simulink model "TwoDegreeFreedom_Model"  (R2019a)
settings: Solver=VariableStepAuto  StartTime=0.0  StopTime=10.0  RelTol=1e-3
undefined symbols (not defined in the file): C_s, K_s, K_t, m_s, m_u
settings Model: Creator=ansar  LastModifiedBy=ansar

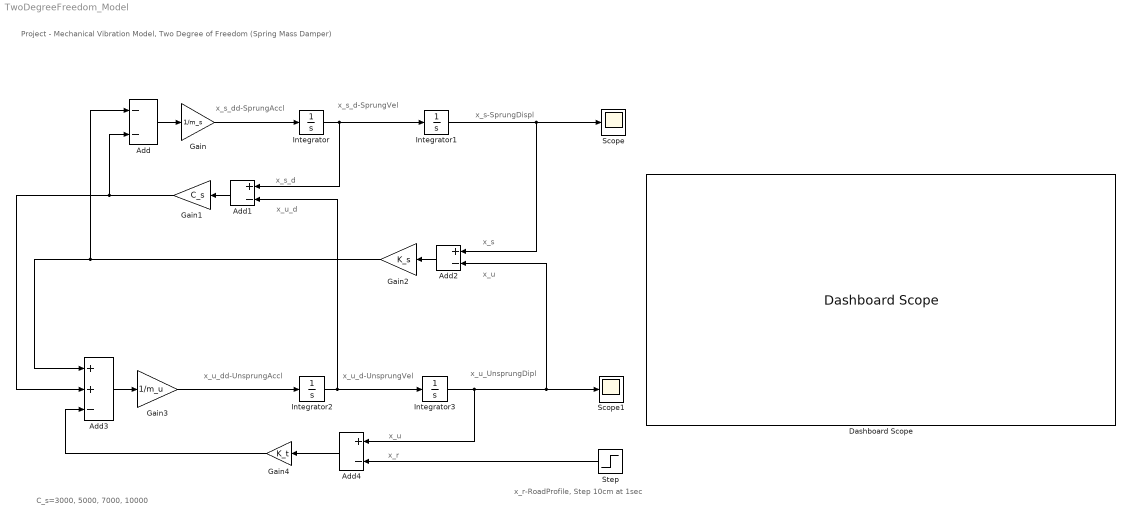
== system TwoDegreeFreedom_Model ==
  note: x_r-RoadProfile, Step 10cm at 1sec
  note: x_r
  note: x_u
  note: x_u
  note: x_s
  note: x_u_d
  note: x_s_d
  note: x_u_UnsprungDipl
  note: x_u_d-UnsprungVel
  note: x_u_dd-UnsprungAccl
  note: x_s-SprungDispl
  note: x_s_d-SprungVel
  note: x_s_dd-SprungAccl
  note: C_s=3000, 5000, 7000, 10000
  note: Project - Mechanical Vibration Model, Two Degree of Freedom (Spring Mass Damper)
  Add : Sum  Inputs=--
  Add1 : Sum  Inputs=+-
  Add2 : Sum  Inputs=+-
  Add3 : Sum  Inputs=++-
  Add4 : Sum  Inputs=+-
  Dashboard Scope : DashboardScope
  Gain : Gain  Gain=1/m_s
  Gain1 : Gain  Gain=C_s
  Gain2 : Gain  Gain=K_s
  Gain3 : Gain  Gain=1/m_u
  Gain4 : Gain  Gain=K_t
  Integrator{,1..3} (4 alike) : Integrator
  Scope : Scope
  Scope1 : Scope
  Step : Step  After=10  SampleTime=0
  wires:
  Gain/1 -> Integrator/1
  Integrator/1 -> Integrator1/1, Add1/1
  Integrator1/1 -> Add2/1, Scope/1
  Add/1 -> Gain/1
  Gain1/1 -> Add3/2, Add/2
  Gain2/1 -> Add3/1, Add/1
  Add1/1 -> Gain1/1
  Add2/1 -> Gain2/1
  Gain3/1 -> Integrator2/1
  Integrator2/1 -> Add1/2, Integrator3/1
  Integrator3/1 -> Add2/2, Scope1/1, Add4/1
  Add3/1 -> Gain3/1
  Gain4/1 -> Add3/3
  Add4/1 -> Gain4/1
  Step/1 -> Add4/2
